simulink model "Droop_control_conditioning_claude"  (R2024b)
settings: Solver=ode4  StartTime=0.0  StopTime=0.4  FixedStep=Ts  RelTol=1e-3
InitFcn:
  | %% ===== Parameters =====================================================
  | %% Every primary parameter is wrapped in ~exist so that a value pushed in
  | %% by Simulink.SimulationInput.setVariable survives this callback. Without
  | %% the guard, InitFcn re-runs at every simulation start and silently
  | %% overwrites the swept value.
  | 
  | %% ---- Droop control ----
  | if ~exist('m1','var'), m1     = 0.5e-5;    end   % f-P droop gain
  | if ~exist('n1','var'), n1     = 5e-3;      end   % Q-V droop gain
  | if ~exist('fn','var'), fn     = 50;        end   % nominal frequency, Hz
  | if ~exist('Vn','var'), Vn     = 325;       end   % nominal voltage, peak
  | if ~exist('wc','var'), wc     = 2*pi*5;    end   % droop low-pass cutoff
  | 
  | %% ---- Voltage controller ----
  | if ~exist('kpv','var'), kpv    = 1;         end   % proportional gain
  | if ~exist('kiv','var'), kiv    = 189;       end   % integral gain
  | if ~exist('F','var'), F      = 0.75;      end   % feedforward gain
  | if ~exist('Ilim1','var'), Ilim1  = 40;        end   % upper limit
  | if ~exist('Ilim2','var'), Ilim2  = -40;       end   % lower limit
  | 
  | %% ---- Current controller ----
  | if ~exist('kpi','var'), kpi    = 10.47*2;   end   % proportional gain
  | if ~exist('kii','var'), kii    = 4188.8*4;  end   % integral gain
  | if ~exist('Vlim1','var'), Vlim1  = 500;       end   % upper limit
  | if ~exist('Vlim2','var'), Vlim2  = 500;       end   % lower limit
  | 
  | %% ---- System parameters ----
  | if ~exist('Lf','var'), Lf     = 1.6e-3;    end   % filter inductance
  | if ~exist('Cf','var'), Cf     = 50e-6;     end   % filter capacitance
  | if ~exist('Rc','var'), Rc     = 0.03;      end   % coupling resistance
  | if ~exist('Lc','var'), Lc     = 0.35e-3;   end   % coupling inductance
  | if ~exist('fs','var'), fs     = 10e3;      end   % switching frequency
  | if ~exist('Ts','var'), Ts     = 10e-7;     end   % solver step - FixedStep follows this
  | if ~exist('Vin','var'), Vin    = 1000;      end   % DC link voltage
  | if ~exist('ts','var'), ts     = 0.04;      end   % black start time
  | Tsample = 20*Ts;                        % derived from Ts, never guarded
  | 
  | %% ---- Line parameters ----
  | if ~exist('R1','var'), R1     = 0.23;      end   % line resistance
  | if ~exist('L1','var'), L1     = 3.1e-4;    end   % line inductance
  | 
  | %% ---- Load bank resistances, per phase, ohm ----
  | %% Bank A: DG1 bus, always connected        (delivered 32 / 32 / 32)
  | %% Bank B: DG1 bus, behind breaker at t=1s  (delivered 160 / 160 / 160)
  | %% Bank C: DG2 bus, always connected        (delivered 160 / 160 / 160)
  | %% Only bank A is swept; B and C stay at their delivered values.
  | if ~exist('R_A_a','var'), R_A_a  = 32;        end   % bank A phase a  <-- swept
  | if ~exist('R_A_b','var'), R_A_b  = 32;        end   % bank A phase b  <-- swept
  | if ~exist('R_A_c','var'), R_A_c  = 32;        end   % bank A phase c  <-- swept
  | if ~exist('R_B_a','var'), R_B_a  = 160;       end   % bank B phase a
  | if ~exist('R_B_b','var'), R_B_b  = 160;       end   % bank B phase b
  | if ~exist('R_B_c','var'), R_B_c  = 160;       end   % bank B phase c
  | if ~exist('R_C_a','var'), R_C_a  = 160;       end   % bank C phase a
  | if ~exist('R_C_b','var'), R_C_b  = 160;       end   % bank C phase b
  | if ~exist('R_C_c','var'), R_C_c  = 160;       end   % bank C phase c
  | 
  | %% ---- PWM pulse masks: 1 = pulse connected, 0 = switch held open ----
  | %% Pulse-to-IGBT mapping is verified empirically by run_pilot.m; see the
  | %% mapping note written there before trusting any per-pulse label.
  | if ~exist('F1','var'), F1     = [1 1 1 1 1 1]; end   % inverter 1  <-- swept
  | ... (+1 lines)
values from neighbouring files (symbols this model uses):
  F1 = [r.DG1_PWM1 r.DG1_PWM2 r.DG1_PWM3 r.DG1_PWM4 r.DG1_PWM5 r.DG1_PWM6]    [run_sweep.m]
  F2 = [r.DG2_PWM1 r.DG2_PWM2 r.DG2_PWM3 r.DG2_PWM4 r.DG2_PWM5 r.DG2_PWM6]    [run_sweep.m]
undefined symbols (not defined in the file or in its folder): Cf, F, fn, Ilim1, Ilim2, kii, kiv, kpi, kpv, L1, Lc, Lf, m1, n1, R1, R_A_a, R_A_b, R_A_c, R_B_a, R_B_b, R_B_c, R_C_a, R_C_b, R_C_c, Rc, ts, Ts, Vin, Vlim1, Vlim2, Vn, wc
libraries: spsSeriesRLCBranchLib x9, slpidlib x8, spsThreePhaseSeriesRLCBranchLib x7, spsabctodq0Lib x6, spsGroundLib x5, spsThreePhaseVIMeasurementLib x5, spsDCVoltageSourceLib x2, spsPowerdq0InstantaneousLib x2, spsPWMGenerator2LevelLib x2, spsUniversalBridgeLib x2, spsdq0toabcLib x2, dspstat3 x1
(part 2 of 2)

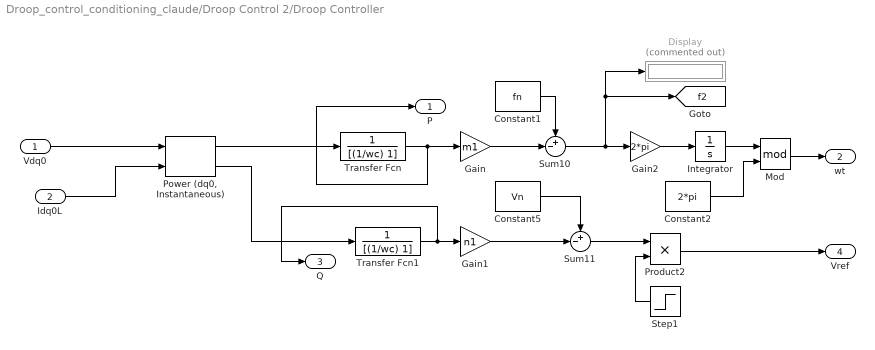
== system Droop_control_conditioning_claude/Droop Control 2/Droop Controller ==
  Vdq0 : Inport
  Idq0L : Inport  Port=2
  Constant1 : Constant  Value=fn
  Constant2 : Constant  Value=2*pi
  Constant5 : Constant  Value=Vn
  Display : Display  Commented=on
  Gain : Gain  Gain=m1
  Gain1 : Gain  Gain=n1
  Gain2 : Gain  Gain=2*pi
  Integrator : Integrator
  Mod : Math  Operator=mod
  "Power (dq0, Instantaneous)" : spsPowerdq0InstantaneousLib/Power (dq0, Instantaneous)
      settings: LibrarySourceBlock=|
      | sps_lib/Sensors and Measurements/Power
      | (dq0, Instantaneous)
  Product2 : Product  Inputs=**
  Step1 : Step  Time=ts  SampleTime=0
  Sum10 : Sum  Inputs=+-|
  Sum11 : Sum  Inputs=+-|
  Transfer Fcn : TransferFcn  Numerator=[0 1]  Denominator=[(1/wc) 1]
  Transfer Fcn1 : TransferFcn  Numerator=[0 1]  Denominator=[(1/wc) 1]
  P : Outport
  wt : Outport  Port=2
  Q : Outport  Port=3
  Vref : Outport  Port=4
  tag scope: f2=global
  wires:
  Sum11/1 -> Product2/1
  Product2/1 -> Vref/1
  Step1/1 -> Product2/2
  Sum10/1 -> Display/1, [f2], Gain2/1
  Gain2/1 -> Integrator/1
  Idq0L/1 -> "Power (dq0, Instantaneous)"/2
  Vdq0/1 -> "Power (dq0, Instantaneous)"/1
  Constant2/1 -> Mod/2
  Mod/1 -> wt/1
  Integrator/1 -> Mod/1
  Transfer Fcn1/1 -> Gain1/1, Q/1
  Transfer Fcn/1 -> Gain/1, P/1
  Gain/1 -> Sum10/2
  Gain1/1 -> Sum11/2
  Constant5/1 -> Sum11/1
  Constant1/1 -> Sum10/1
  "Power (dq0, Instantaneous)"/1 -> Transfer Fcn/1
  "Power (dq0, Instantaneous)"/2 -> Transfer Fcn1/1

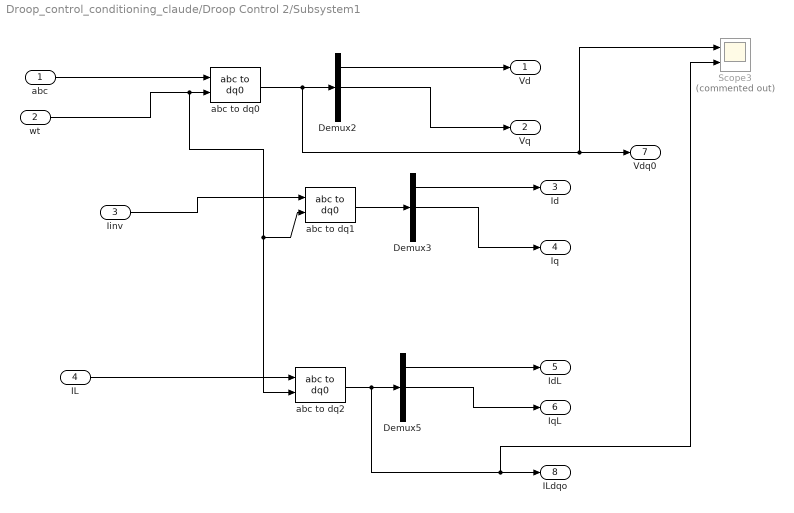
== system Droop_control_conditioning_claude/Droop Control 2/Subsystem1 ==
  abc : Inport
  wt : Inport  Port=2
  Iinv : Inport  Port=3
  IL : Inport  Port=4
  Demux2 : Demux  Outputs=3
  Demux3 : Demux  Outputs=3
  Demux5 : Demux  Outputs=3
  Scope3 : Scope  Commented=on  NumInputPorts=2
  abc to dq0 : spsabctodq0Lib/abc to dq0  Alignment=90 degrees behind phase A axis
  abc to dq1 : spsabctodq0Lib/abc to dq0  Alignment=90 degrees behind phase A axis
  abc to dq2 : spsabctodq0Lib/abc to dq0  Alignment=90 degrees behind phase A axis
  Vd : Outport
  Vq : Outport  Port=2
  Id : Outport  Port=3
  Iq : Outport  Port=4
  IdL : Outport  Port=5
  IqL : Outport  Port=6
  Vdq0 : Outport  Port=7
  ILdqo : Outport  Port=8
  wires:
  IL/1 -> abc to dq2/1
  Demux3/2 -> Iq/1
  abc/1 -> abc to dq0/1
  Demux5/2 -> IqL/1
  Demux5/1 -> IdL/1
  Demux2/1 -> Vd/1
  Demux3/1 -> Id/1
  Iinv/1 -> abc to dq1/1
  Demux2/2 -> Vq/1
  wt/1 -> abc to dq0/2, abc to dq1/2, abc to dq2/2
  abc to dq1/1 -> Demux3/1
  abc to dq2/1 -> Demux5/1, ILdqo/1, Scope3/2
  abc to dq0/1 -> Demux2/1, Vdq0/1, Scope3/1

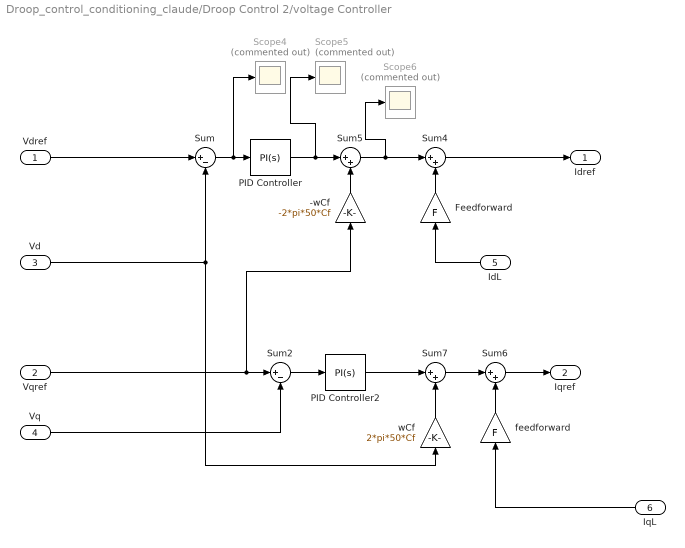
== system Droop_control_conditioning_claude/Droop Control 2/voltage Controller ==
  Vdref : Inport
  Vqref : Inport  Port=2
  Vd : Inport  Port=3
  Vq : Inport  Port=4
  IdL : Inport  Port=5
  IqL : Inport  Port=6
  -wCf : Gain  Gain=-2*pi*50*Cf
  Feedforward : Gain  Gain=F
  PID Controller : slpidlib/PID Controller  Controller=PI  Form=Parallel  TimeDomain=Continuous-time  UseExternalTs=off  SampleTime=Tsample  IntegratorMethod=Forward Euler  FilterMethod=Forward Euler  ControllerParametersSource=internal  P=kpv  I=kiv  UseKiTs=off  D=0  UseExternalDerivativeSource=off  N=100  UseFilter=on  TunerSelectOption=Transfer Function Based (PID Tuner App)  InitialConditionSource=internal  InitialConditionForIntegrator=0  InitialConditionForFilter=0  DifferentiatorICPrevScaledInput=0  ExternalReset=none  TrackingMode=off  Kt=1  LimitOutput=off  SatLimitsSource=internal  UpperSaturationLimit=Vlim1  LowerSaturationLimit=Vlim2  LinearizeAsGain=off  AntiWindupMode=none  Kb=1  LimitIntegrator=off  UpperIntegratorSaturationLimit=inf  LowerIntegratorSaturationLimit=-inf  POutMin=[]  POutMax=[]  IOutMin=[]  IOutMax=[]  DOutMin=[]  DOutMax=[]  NOutMin=[]  NOutMax=[]  SumOutMin=[]  SumOutMax=[]  SaturationOutMin=[]  SaturationOutMax=[]  PParamMin=[]  PParamMax=[]  IParamMin=[]  IParamMax=[]  DParamMin=[]  DParamMax=[]  NParamMin=[]  NParamMax=[]  KbParamMin=[]  KbParamMax=[]  KtParamMin=[]  KtParamMax=[]  KbOutMin=[]  KbOutMax=[]  KtOutMin=[]  KtOutMax=[]  IntegratorOutMin=[]  IntegratorOutMax=[]  FilterOutMin=[]  FilterOutMax=[]  SumI1OutMin=[]  SumI1OutMax=[]  SumI2OutMin=[]  SumI2OutMax=[]  SumI3OutMin=[]  SumI3OutMax=[]  SumI4OutMin=[]  SumI4OutMax=[]  SumDOutMin=[]  SumDOutMax=[]  DifferentiatorOutMin=[]  DifferentiatorOutMax=[]  FilterDiffOutCoefMin=[]  FilterDiffOutCoefMax=[]  ReciprocalOutMin=[]  ReciprocalOutMax=[]  SumDenOutMin=[]  SumDenOutMax=[]  SumNumOutMin=[]  SumNumOutMax=[]  DivideOutMin=[]  DivideOutMax=[]  UdiffTsProdOutMin=[]  UdiffTsProdOutMax=[]  NTsProdOutMin=[]  NTsProdOutMax=[]  UintegralTsProdOutMin=[]  UintegralTsProdOutMax=[]  UngainTsProdOutMin=[]  UngainTsProdOutMax=[]  ClampingZeroOutDataTypeStr=Inherit: Inherit via back propagation  ClampingZeroOutMin=[]  ClampingZeroOutMax=[]  FilterDenConstantOutDataTypeStr=Inherit: Inherit via back propagation  FilterDenConstantOutMin=[]  FilterDenConstantOutMax=[]  PCopyOutDataTypeStr=Inherit: Inherit via back propagation  PCopyOutMin=[]  PCopyOutMax=[]  NCopyOutDataTypeStr=Inherit: Inherit via back propagation  NCopyOutMin=[]  NCopyOutMax=[]  IntegratorContinuousStateAttributes=''  IntegratorStateMustResolveToSignalObject=off  IntegratorRTWStateStorageClass=Auto  FilterContinuousStateAttributes=''  FilterStateMustResolveToSignalObject=off  FilterRTWStateStorageClass=Auto  ParallelPVariant=InternalParameters  IdealPVariant=Disabled  IVariant=InternalParameters  DVariant=Disabled  IntegratorVariant=Continuous  SatVariant=Disabled  AWVariant=Passthrough  PCopyVariant=Disabled  TRVariant=Disabled  FdbkBlocksVariant=Forward  IdealPFdbkVariant=Disabled  SatFdbkVariant=Disabled  DerivativeFilterVariant=Disabled  NVariant=Disabled  NCopyVariant=Disabled_SignalSpec  FilterICVariant=Disabled  IntegratorICVariant=InternalICs  ExternalResetVariant=Disabled  TRSumVariant=Passthrough  SumFdbkVariant=Disabled  SumVariant=Sum_PI  TsampFilterVariant=InternalTs  TsampNgainVariant=Passthrough  TsampIntegralVariant=Disabled_SignalSpec  ExternalSaturationOutDataTypeStr=Inherit: Same as second input  DerivativeSourceVariant=Disabled  PreIntVariant=InternalPreInt
  PID Controller2 : slpidlib/PID Controller  Controller=PI  Form=Parallel  TimeDomain=Continuous-time  UseExternalTs=off  SampleTime=Tsample  IntegratorMethod=Forward Euler  FilterMethod=Forward Euler  ControllerParametersSource=internal  P=kpv  I=kiv  UseKiTs=off  D=0  UseExternalDerivativeSource=off  N=100  UseFilter=on  TunerSelectOption=Transfer Function Based (PID Tuner App)  InitialConditionSource=internal  InitialConditionForIntegrator=0  InitialConditionForFilter=0  DifferentiatorICPrevScaledInput=0  ExternalReset=none  TrackingMode=off  Kt=1  LimitOutput=off  SatLimitsSource=internal  UpperSaturationLimit=Vlim1  LowerSaturationLimit=Vlim2  LinearizeAsGain=off  AntiWindupMode=none  Kb=1  LimitIntegrator=off  UpperIntegratorSaturationLimit=inf  LowerIntegratorSaturationLimit=-inf  POutMin=[]  POutMax=[]  IOutMin=[]  IOutMax=[]  DOutMin=[]  DOutMax=[]  NOutMin=[]  NOutMax=[]  SumOutMin=[]  SumOutMax=[]  SaturationOutMin=[]  SaturationOutMax=[]  PParamMin=[]  PParamMax=[]  IParamMin=[]  IParamMax=[]  DParamMin=[]  DParamMax=[]  NParamMin=[]  NParamMax=[]  KbParamMin=[]  KbParamMax=[]  KtParamMin=[]  KtParamMax=[]  KbOutMin=[]  KbOutMax=[]  KtOutMin=[]  KtOutMax=[]  IntegratorOutMin=[]  IntegratorOutMax=[]  FilterOutMin=[]  FilterOutMax=[]  SumI1OutMin=[]  SumI1OutMax=[]  SumI2OutMin=[]  SumI2OutMax=[]  SumI3OutMin=[]  SumI3OutMax=[]  SumI4OutMin=[]  SumI4OutMax=[]  SumDOutMin=[]  SumDOutMax=[]  DifferentiatorOutMin=[]  DifferentiatorOutMax=[]  FilterDiffOutCoefMin=[]  FilterDiffOutCoefMax=[]  ReciprocalOutMin=[]  ReciprocalOutMax=[]  SumDenOutMin=[]  SumDenOutMax=[]  SumNumOutMin=[]  SumNumOutMax=[]  DivideOutMin=[]  DivideOutMax=[]  UdiffTsProdOutMin=[]  UdiffTsProdOutMax=[]  NTsProdOutMin=[]  NTsProdOutMax=[]  UintegralTsProdOutMin=[]  UintegralTsProdOutMax=[]  UngainTsProdOutMin=[]  UngainTsProdOutMax=[]  ClampingZeroOutDataTypeStr=Inherit: Inherit via back propagation  ClampingZeroOutMin=[]  ClampingZeroOutMax=[]  FilterDenConstantOutDataTypeStr=Inherit: Inherit via back propagation  FilterDenConstantOutMin=[]  FilterDenConstantOutMax=[]  PCopyOutDataTypeStr=Inherit: Inherit via back propagation  PCopyOutMin=[]  PCopyOutMax=[]  NCopyOutDataTypeStr=Inherit: Inherit via back propagation  NCopyOutMin=[]  NCopyOutMax=[]  IntegratorContinuousStateAttributes=''  IntegratorStateMustResolveToSignalObject=off  IntegratorRTWStateStorageClass=Auto  FilterContinuousStateAttributes=''  FilterStateMustResolveToSignalObject=off  FilterRTWStateStorageClass=Auto  ParallelPVariant=InternalParameters  IdealPVariant=Disabled  IVariant=InternalParameters  DVariant=Disabled  IntegratorVariant=Continuous  SatVariant=Disabled  AWVariant=Passthrough  PCopyVariant=Disabled  TRVariant=Disabled  FdbkBlocksVariant=Forward  IdealPFdbkVariant=Disabled  SatFdbkVariant=Disabled  DerivativeFilterVariant=Disabled  NVariant=Disabled  NCopyVariant=Disabled_SignalSpec  FilterICVariant=Disabled  IntegratorICVariant=InternalICs  ExternalResetVariant=Disabled  TRSumVariant=Passthrough  SumFdbkVariant=Disabled  SumVariant=Sum_PI  TsampFilterVariant=InternalTs  TsampNgainVariant=Passthrough  TsampIntegralVariant=Disabled_SignalSpec  ExternalSaturationOutDataTypeStr=Inherit: Same as second input  DerivativeSourceVariant=Disabled  PreIntVariant=InternalPreInt
  Scope4 : Scope  Commented=on
  Scope5 : Scope  Commented=on
  Scope6 : Scope  Commented=on
  Sum : Sum  Inputs=|+-
  Sum2 : Sum  Inputs=|+-
  Sum{4..7} (4 alike) : Sum  Inputs=|++
  feedforward : Gain  Gain=F
  wCf : Gain  Gain=2*pi*50*Cf
  Idref : Outport
  Iqref : Outport  Port=2
  wires:
  IdL/1 -> Feedforward/1
  Vqref/1 -> Sum2/1, -wCf/1
  PID Controller/1 -> Sum5/1, Scope5/1
  Vdref/1 -> Sum/1
  -wCf/1 -> Sum5/2
  Sum2/1 -> PID Controller2/1
  wCf/1 -> Sum7/2
  Feedforward/1 -> Sum4/2
  Sum6/1 -> Iqref/1
  PID Controller2/1 -> Sum7/1
  Vq/1 -> Sum2/2
  Vd/1 -> wCf/1, Sum/2
  IqL/1 -> feedforward/1
  Sum7/1 -> Sum6/1
  feedforward/1 -> Sum6/2
  Sum5/1 -> Sum4/1, Scope6/1
  Sum/1 -> PID Controller/1, Scope4/1
  Sum4/1 -> Idref/1
